simulink model "Hw2Pr2"  (Simulink 7.2)
settings: Solver=ode45  StartTime=0.0  StopTime=5  RelTol=1e-3
libraries: roblocks x1
settings Model: Creator=Chris  LastModifiedBy=Chris
settings DataIOCC: SignalLoggingName=sigsOut
settings DebuggingCC: SaveWithParameterizedLinksMsg=none  SignalResolutionControl=TryResolveAllWithWarning  SolverPrmCheckMsg=none  MultiTaskDSMMsg=warning  MultiTaskCondExecSysMsg=none  StrictBusMsg=None
settings HardwareCC: TargetUnknown=on
settings RTWCC: IncludeERTFirstTime=on

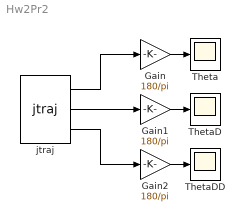
== system Hw2Pr2 ==
  Gain : Gain  Gain=180/pi  ParameterDataType=sfix(16)  ParameterScaling=2^0  OutDataType=sfix(16)  OutScaling=2^0  SaturateOnIntegerOverflow=on  OutDataTypeStr=Inherit: Same as input  ParamDataTypeStr=Inherit: Same as input
  Gain1 : Gain  Gain=180/pi  ParameterDataType=sfix(16)  ParameterScaling=2^0  OutDataType=sfix(16)  OutScaling=2^0  SaturateOnIntegerOverflow=on  OutDataTypeStr=Inherit: Same as input  ParamDataTypeStr=Inherit: Same as input
  Gain2 : Gain  Gain=180/pi  ParameterDataType=sfix(16)  ParameterScaling=2^0  OutDataType=sfix(16)  OutScaling=2^0  SaturateOnIntegerOverflow=on  OutDataTypeStr=Inherit: Same as input  ParamDataTypeStr=Inherit: Same as input
  Theta : Scope
  ThetaD : Scope
  ThetaDD : Scope
      settings: SaveName=ScopeData2
  jtraj : roblocks/jtraj  SystemSampleTime=-1  q0=[-pi/3]  qf=[pi/3]  tmax=5
  wires:
  Gain/1 -> Theta/1
  Gain2/1 -> ThetaDD/1
  Gain1/1 -> ThetaD/1
  jtraj/2 -> Gain1/1
  jtraj/1 -> Gain/1
  jtraj/3 -> Gain2/1
